simulink model "MotorCntrl"  (R2020b)
settings: Solver=VariableStepAuto  StartTime=0.0  StopTime=10.0  RelTol=1e-3
settings Model: DataDictionary=Motor_DataDictionary.sldd  Creator=Sourav Kumar  LastModifiedBy=Sourav Kumar

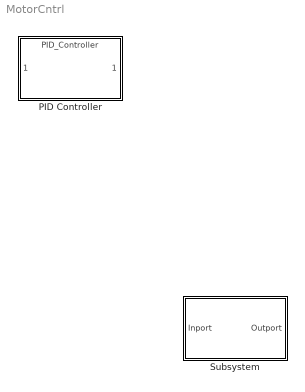
== system MotorCntrl ==
  PID Controller : ModelReference  ModelNameDialog=PID_Controller  SimulationMode=Normal  ModelReferenceVersion=1.4
  Subsystem : Subsystem

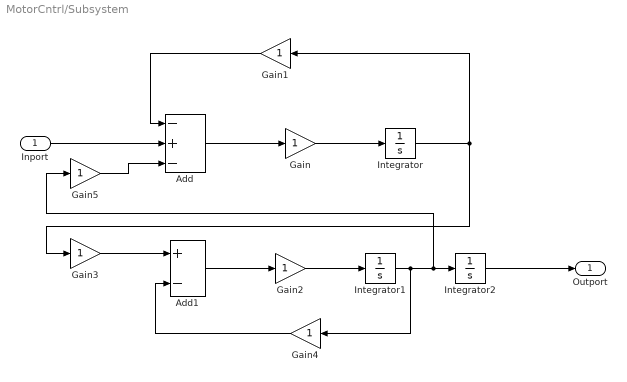
== system MotorCntrl/Subsystem ==
  Inport : Inport
  Add : Sum  Inputs=-+-
  Add1 : Sum  Inputs=+-
  Gain{,1..5} (6 alike) : Gain
  Integrator : Integrator
  Integrator1 : Integrator
  Integrator2 : Integrator
  Outport : Outport
  wires:
  Integrator1/1 -> Gain4/1, Gain5/1, Integrator2/1
  Add/1 -> Gain/1
  Gain/1 -> Integrator/1
  Integrator/1 -> Gain3/1, Gain1/1
  Gain1/1 -> Add/1
  Inport/1 -> Add/2
  Add1/1 -> Gain2/1
  Integrator2/1 -> Outport/1
  Gain4/1 -> Add1/2
  Gain5/1 -> Add/3
  Gain2/1 -> Integrator1/1
  Gain3/1 -> Add1/1
